simulink model "mavsim_DemoTrimStates"  (R2015a)
settings: Solver=ode45  StartTime=0.0  StopTime=10000  RelTol=1e-3
undefined symbols (not defined in the file or in its folder): drawAircraft, forces_moments, P, plotmavstatevariables
libraries: simulink x4
settings Model: CovSFcnEnable=off  Creator=beard  LastModifiedBy=Scott
settings DataIOCC: SignalLoggingSaveFormat=ModelDataLogs
settings OptimizationCC: ExpressionDepthLimit=2147483647  InitFltsAndDblsToZero=on
settings DebuggingCC: UnderspecifiedInitializationDetection=Classic  MergeDetectMultiDrivingBlocksExec=none  SolverPrmCheckMsg=warning  FcnCallInpInsideContextMsg=UseLocalSettings  StateNameClashWarn=warning
settings GRTTargetCC: CombineOutputUpdateFcns=off  GRTInterface=on

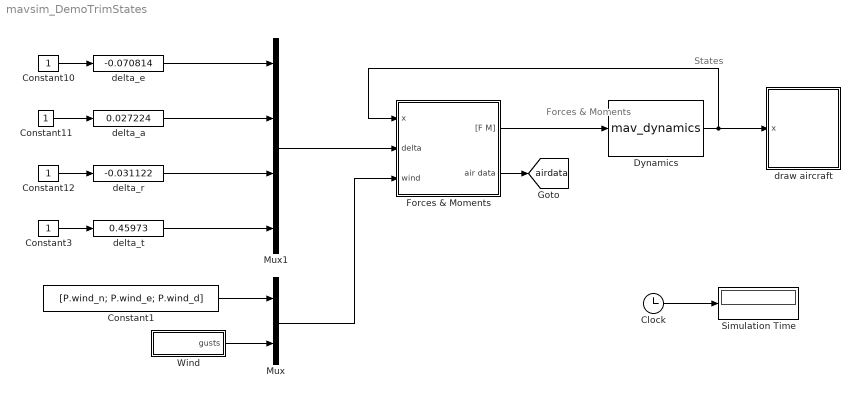
== system mavsim_DemoTrimStates ==
  note: Forces & Moments
  note: States
  Clock : Clock
  Constant1 : Constant  Value=[P.wind_n; P.wind_e; P.wind_d]
  Constant{3,10..12} (4 alike) : Constant
  Dynamics : S-Function  FunctionName=mav_dynamics  Parameters=P
  Forces & Moments : Subsystem
  Mux : Mux  Inputs=2
  Mux1 : Mux
  Simulation Time : Display
  Wind : Subsystem
  delta_a : simulink/Math Operations/Slider Gain  low=-45  gain=0.027224  high=45
  delta_e : simulink/Math Operations/Slider Gain  low=-45  gain=-0.070814  high=45
  delta_r : simulink/Math Operations/Slider Gain  low=-45  gain=-0.031122  high=45
  delta_t : simulink/Math Operations/Slider Gain  low=0  gain=0.45973  high=1
  draw aircraft : Subsystem
      mask Display: image(imread('tv.jpg'))
  tag scope: airdata=global
  wires:
  Constant10/1 -> delta_e/1
  Constant11/1 -> delta_a/1
  Constant12/1 -> delta_r/1
  Dynamics/1 -> draw aircraft/1(x), Forces & Moments/1(x)
  Constant3/1 -> delta_t/1
  delta_t/1 -> Mux1/4
  Mux1/1 -> Forces & Moments/2(delta)
  Forces & Moments/1("[F M]") -> Dynamics/1
  Clock/1 -> Simulation Time/1
  Mux/1 -> Forces & Moments/3(wind)
  Constant1/1 -> Mux/1
  Forces & Moments/2(air data) -> [airdata]
  delta_r/1 -> Mux1/3
  delta_e/1 -> Mux1/1
  delta_a/1 -> Mux1/2
  Wind/1(gusts) -> Mux/2

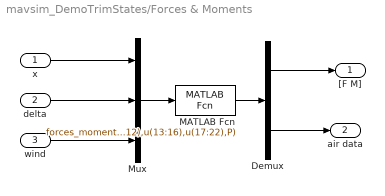
== system mavsim_DemoTrimStates/Forces & Moments ==
  x : Inport
  delta : Inport  Port=2
  wind : Inport  Port=3
  Demux : Demux  Outputs=[6;6]
  MATLAB Fcn : MATLABFcn  MATLABFcn=forces_moments(u(1:12),u(13:16),u(17:22),P)  OutputDimensions=12
  Mux : Mux  Inputs=3
  "[F M]" : Outport
  air data : Outport  Port=2
  wires:
  x/1 -> Mux/1
  delta/1 -> Mux/2
  wind/1 -> Mux/3
  MATLAB Fcn/1 -> Demux/1
  Demux/1 -> "[F M]"/1
  Mux/1 -> MATLAB Fcn/1
  Demux/2 -> air data/1

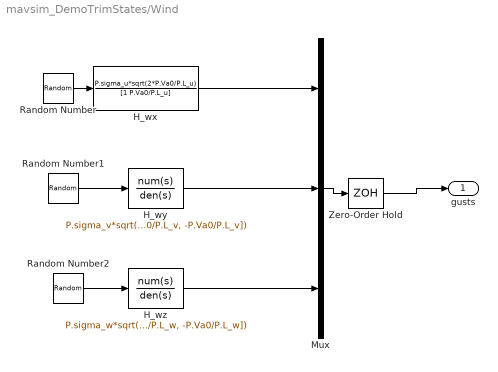
== system mavsim_DemoTrimStates/Wind ==
  H_wx : TransferFcn  Numerator=P.sigma_u*sqrt(2*P.Va0/P.L_u)  Denominator=[1 P.Va0/P.L_u]
  H_wy : TransferFcn  Numerator=P.sigma_v*sqrt(3*P.Va0/P.L_v)*[0, 1, P.Va0/sqrt(3)/P.L_v]  Denominator=poly([-P.Va0/P.L_v, -P.Va0/P.L_v])
  H_wz : TransferFcn  Numerator=P.sigma_w*sqrt(3*P.Va0/P.L_w)*[0, 1, P.Va0/sqrt(3)/P.L_w]  Denominator=poly([-P.Va0/P.L_w, -P.Va0/P.L_w])
  Mux : Mux  Inputs=3
  Random Number : RandomNumber  SampleTime=0
  Random Number1 : RandomNumber  SampleTime=0
  Random Number2 : RandomNumber  SampleTime=0
  Zero-Order Hold : ZeroOrderHold  SampleTime=P.Ts
  gusts : Outport
  wires:
  H_wx/1 -> Mux/1
  Random Number/1 -> H_wx/1
  H_wy/1 -> Mux/2
  Random Number1/1 -> H_wy/1
  H_wz/1 -> Mux/3
  Random Number2/1 -> H_wz/1
  Mux/1 -> Zero-Order Hold/1
  Zero-Order Hold/1 -> gusts/1

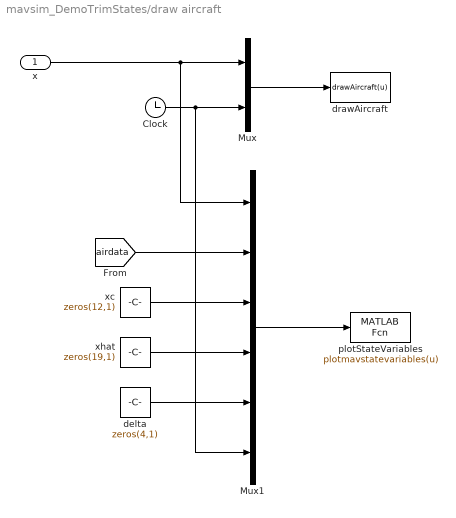
== system mavsim_DemoTrimStates/draw aircraft ==
  x : Inport
  Clock : Clock
  Mux : Mux  Inputs=2
  Mux1 : Mux  Inputs=6
  delta : Constant  Value=zeros(4,1)
  drawAircraft : MATLABFcn  MATLABFcn=drawAircraft(u)  OutputDimensions=0  SampleTime=0.1
  plotStateVariables : MATLABFcn  MATLABFcn=plotmavstatevariables(u)  OutputDimensions=0  SampleTime=0.1
  xc : Constant  Value=zeros(12,1)
  xhat : Constant  Value=zeros(19,1)
  wires:
  delta/1 -> Mux1/5
  xc/1 -> Mux1/3
  xhat/1 -> Mux1/4
  Mux1/1 -> plotStateVariables/1
  Clock/1 -> Mux1/6, Mux/2
  x/1 -> Mux1/1, Mux/1
  Mux/1 -> drawAircraft/1
  [airdata] -> Mux1/2
